simulink model "Controller_ETR"  (R2013b)
settings: Solver=ode45  StartTime=0.0  StopTime=10.0  RelTol=1e-3
undefined symbols (not defined in the file or in its folder): K_dot_track, K_dot_wait, K_track, K_wait
libraries: dspvision x1
settings Model: Creator=hkunte  LastModifiedBy=menkh

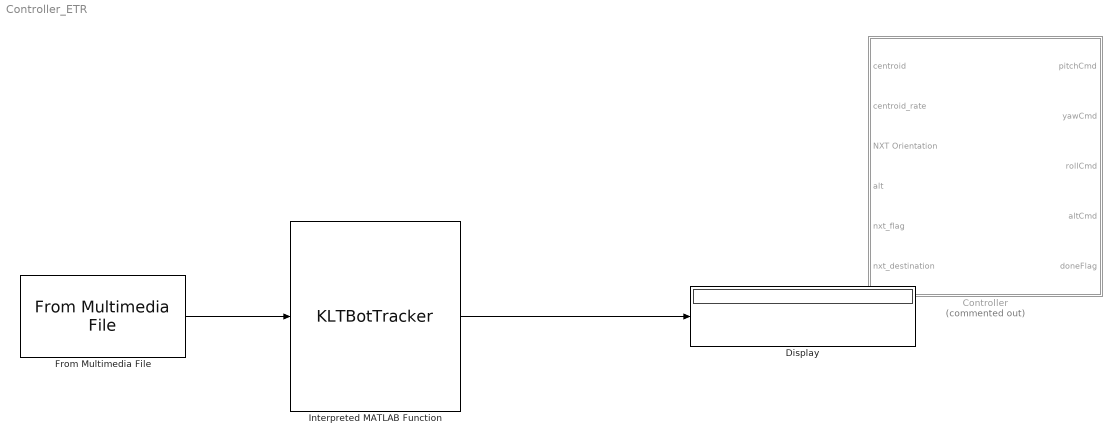
== system Controller_ETR ==
  "Controller " : Subsystem  Commented=on
  Display : Display
  From Multimedia File : dspvision/From Multimedia File  inputFilename=natickTrial7.mp4  loop=on  numPlays=inf  outputStreams=Video only  videoDataType=double  audioDataType=int16  inheritSampleTime=on  userDefinedSampleTime=1/30  noAudioOutput=off  isIntensityVideo=off  fourcc=Intensity  colorVideoFormat=Separate color signals  outputEOF=off  dataOrg=Column-major  audioFrameSize=1024  computeAudioFrameSize=off  outSamplingMode=Sample based
  Interpreted MATLAB Function : MATLABFcn  MATLABFcn=KLTBotTracker  OutputDimensions=[1 2]  Output1D=off
  wires:
  Interpreted MATLAB Function/1 -> Display/1
  From Multimedia File/1 -> Interpreted MATLAB Function/1

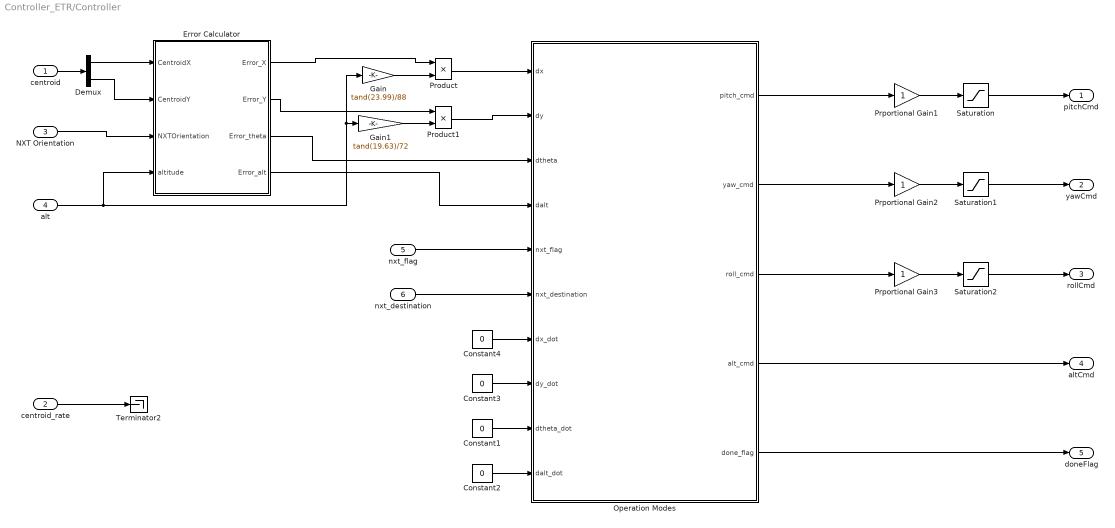
== system Controller_ETR/Controller  ==
  centroid : Inport
  "centroid_rate " : Inport  Port=2  PortDimensions=2
  NXT Orientation : Inport  Port=3
  alt : Inport  Port=4
  nxt_flag : Inport  Port=5  OutDataTypeStr=boolean
  nxt_destination : Inport  Port=6  OutDataTypeStr=boolean
  Constant{1..4} (4 alike) : Constant  Value=0
  Demux : Demux  Outputs=2
  Error Calculator : Subsystem
  Gain : Gain  Gain=tand(23.99)/88
  Gain1 : Gain  Gain=tand(19.63)/72
  Operation Modes : Stateflow chart  TreatAsAtomicUnit=on
  Product : Product
  Product1 : Product
  Prportional Gain1 : Gain
  Prportional Gain2 : Gain
  Prportional Gain3 : Gain
  Saturation : Saturate  UpperLimit=1  LowerLimit=-1
  Saturation1 : Saturate  UpperLimit=1  LowerLimit=-1
  Saturation2 : Saturate  UpperLimit=1  LowerLimit=-1
  Terminator2 : Terminator
  pitchCmd : Outport
  yawCmd : Outport  Port=2
  rollCmd : Outport  Port=3
  altCmd : Outport  Port=4
  doneFlag : Outport  Port=5
  wires:
  Constant2/1 -> Operation Modes/10(dalt_dot)
  Demux/2 -> Error Calculator/2(CentroidY)
  Demux/1 -> Error Calculator/1(CentroidX)
  centroid/1 -> Demux/1
  Saturation1/1 -> yawCmd/1
  Prportional Gain3/1 -> Saturation2/1
  Operation Modes/1(pitch_cmd) -> Prportional Gain1/1
  Saturation2/1 -> rollCmd/1
  Prportional Gain2/1 -> Saturation1/1
  Prportional Gain1/1 -> Saturation/1
  Operation Modes/3(roll_cmd) -> Prportional Gain3/1
  Saturation/1 -> pitchCmd/1
  Operation Modes/2(yaw_cmd) -> Prportional Gain2/1
  Constant3/1 -> Operation Modes/8(dy_dot)
  Constant1/1 -> Operation Modes/9(dtheta_dot)
  Error Calculator/3(Error_theta) -> Operation Modes/3(dtheta)
  Constant4/1 -> Operation Modes/7(dx_dot)
  Product1/1 -> Operation Modes/2(dy)
  Error Calculator/2(Error_Y) -> Product1/1
  Error Calculator/1(Error_X) -> Product/1
  Product/1 -> Operation Modes/1(dx)
  NXT Orientation/1 -> Error Calculator/3(NXTOrientation)
  alt/1 -> Error Calculator/4(altitude), Gain/1, Gain1/1
  Gain/1 -> Product/2
  Gain1/1 -> Product1/2
  nxt_flag/1 -> Operation Modes/5(nxt_flag)
  "centroid_rate "/1 -> Terminator2/1
  nxt_destination/1 -> Operation Modes/6(nxt_destination)
  Operation Modes/5(done_flag) -> doneFlag/1
  Operation Modes/4(alt_cmd) -> altCmd/1
  Error Calculator/4(Error_alt) -> Operation Modes/4(dalt)

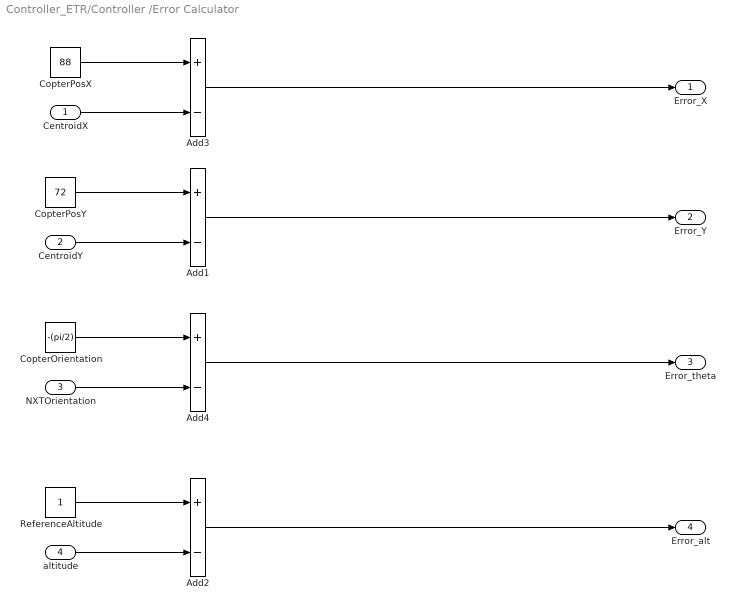
== system Controller_ETR/Controller /Error Calculator ==
  CentroidX : Inport
  CentroidY : Inport  Port=2
  NXTOrientation : Inport  Port=3
  altitude : Inport  Port=4
  Add{1..4} (4 alike) : Sum  Inputs=+-
  CopterOrientation : Constant  Value=-(pi/2)
  CopterPosX : Constant  Value=88
  CopterPosY : Constant  Value=72
  ReferenceAltitude : Constant
  Error_X : Outport
  Error_Y : Outport  Port=2
  Error_theta : Outport  Port=3
  Error_alt : Outport  Port=4
  wires:
  CopterPosY/1 -> Add1/1
  CentroidY/1 -> Add1/2
  CopterPosX/1 -> Add3/1
  CentroidX/1 -> Add3/2
  Add3/1 -> Error_X/1
  Add1/1 -> Error_Y/1
  NXTOrientation/1 -> Add4/2
  CopterOrientation/1 -> Add4/1
  Add4/1 -> Error_theta/1
  ReferenceAltitude/1 -> Add2/1
  altitude/1 -> Add2/2
  Add2/1 -> Error_alt/1

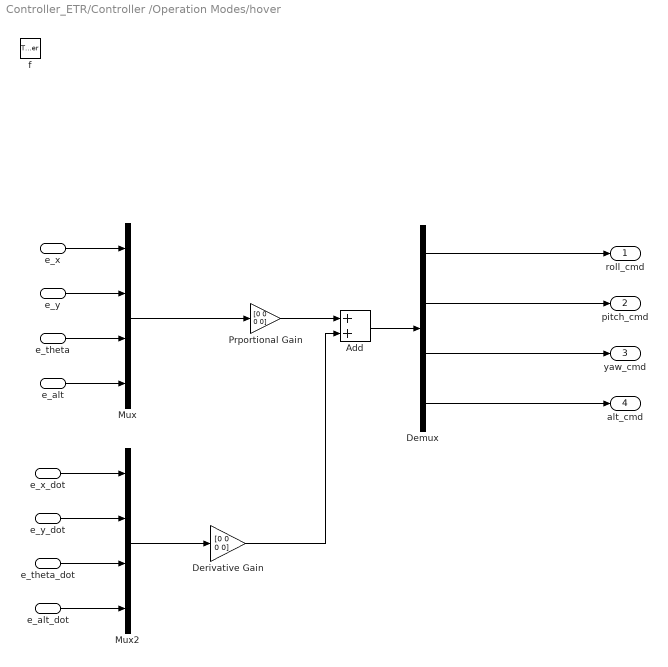
== system Controller_ETR/Controller /Operation Modes/hover ==
  e_x : Inport
  e_y : Inport  Port=2
  e_theta : Inport  Port=3
  e_x_dot : Inport  Port=4
  e_y_dot : Inport  Port=5
  e_theta_dot : Inport  Port=6
  e_alt : Inport  Port=7
  e_alt_dot : Inport  Port=8
  f : TriggerPort  TriggerType=function-call
      settings: CopyFcn=Stateflow.SLINSF.SimulinkMan.removeBlockPreDeleteFcn  PreDeleteFcn=Stateflow.SLINSF.SimulinkMan.unsafePredeleteFcn
  Add : Sum
  Demux : Demux
  Derivative Gain : Gain  Gain=[0 0 0 0]
  Mux : Mux
  Mux2 : Mux
  Prportional Gain : Gain  Gain=[0 0 0 0]
  roll_cmd : Outport
  pitch_cmd : Outport  Port=2
  yaw_cmd : Outport  Port=3
  alt_cmd : Outport  Port=4
  wires:
  Mux/1 -> Prportional Gain/1
  e_x/1 -> Mux/1
  e_y/1 -> Mux/2
  e_theta/1 -> Mux/3
  Prportional Gain/1 -> Add/1
  Derivative Gain/1 -> Add/2
  Add/1 -> Demux/1
  Demux/3 -> yaw_cmd/1
  Demux/1 -> roll_cmd/1
  Demux/2 -> pitch_cmd/1
  Mux2/1 -> Derivative Gain/1
  e_x_dot/1 -> Mux2/1
  e_y_dot/1 -> Mux2/2
  e_theta_dot/1 -> Mux2/3
  e_alt/1 -> Mux/4
  e_alt_dot/1 -> Mux2/4
  Demux/4 -> alt_cmd/1

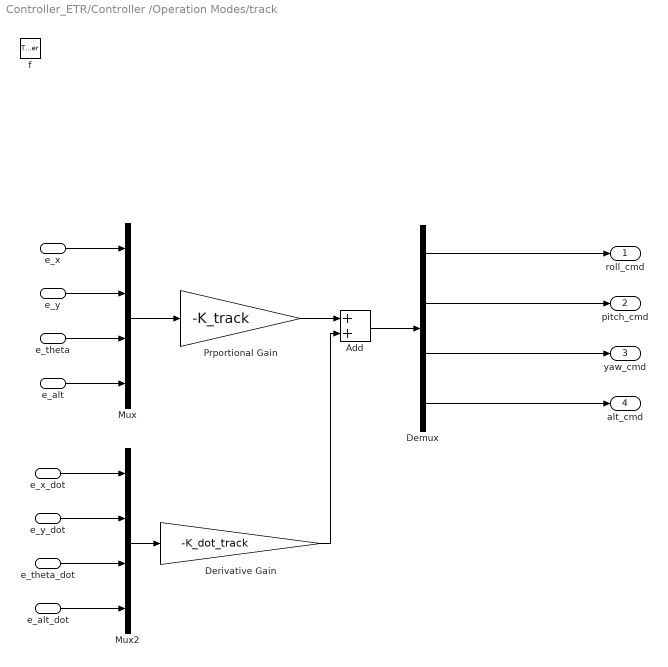
== system Controller_ETR/Controller /Operation Modes/track ==
  e_x : Inport
  e_y : Inport  Port=2
  e_theta : Inport  Port=3
  e_x_dot : Inport  Port=4
  e_y_dot : Inport  Port=5
  e_theta_dot : Inport  Port=6
  e_alt : Inport  Port=7
  e_alt_dot : Inport  Port=8
  f : TriggerPort  TriggerType=function-call
      settings: CopyFcn=Stateflow.SLINSF.SimulinkMan.removeBlockPreDeleteFcn  PreDeleteFcn=Stateflow.SLINSF.SimulinkMan.unsafePredeleteFcn
  Add : Sum
  Demux : Demux
  Derivative Gain : Gain  Gain=-K_dot_track
  Mux : Mux
  Mux2 : Mux
  Prportional Gain : Gain  Gain=-K_track
  roll_cmd : Outport
  pitch_cmd : Outport  Port=2
  yaw_cmd : Outport  Port=3
  alt_cmd : Outport  Port=4
  wires:
  Mux/1 -> Prportional Gain/1
  e_x/1 -> Mux/1
  e_y/1 -> Mux/2
  e_theta/1 -> Mux/3
  Prportional Gain/1 -> Add/1
  Derivative Gain/1 -> Add/2
  Add/1 -> Demux/1
  Demux/3 -> yaw_cmd/1
  Demux/1 -> roll_cmd/1
  Demux/2 -> pitch_cmd/1
  Mux2/1 -> Derivative Gain/1
  e_x_dot/1 -> Mux2/1
  e_y_dot/1 -> Mux2/2
  e_theta_dot/1 -> Mux2/3
  e_alt/1 -> Mux/4
  e_alt_dot/1 -> Mux2/4
  Demux/4 -> alt_cmd/1

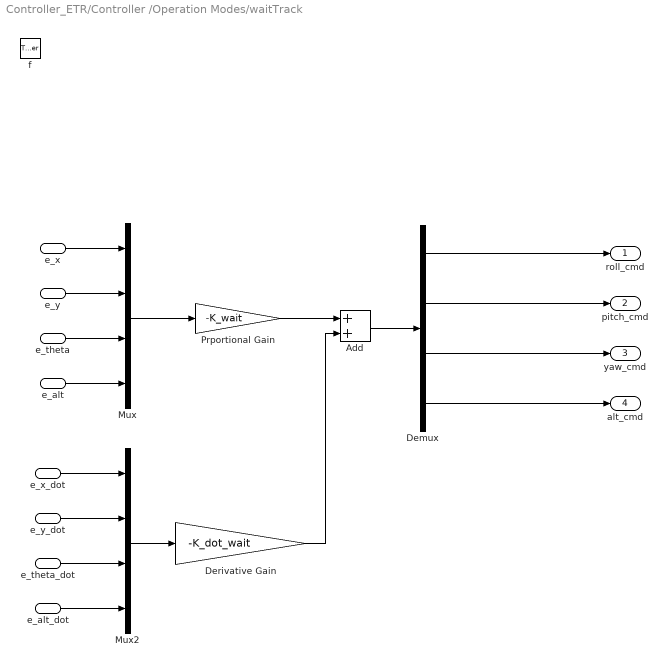
== system Controller_ETR/Controller /Operation Modes/waitTrack ==
  e_x : Inport
  e_y : Inport  Port=2
  e_theta : Inport  Port=3
  e_x_dot : Inport  Port=4
  e_y_dot : Inport  Port=5
  e_theta_dot : Inport  Port=6
  e_alt : Inport  Port=7
  e_alt_dot : Inport  Port=8
  f : TriggerPort  TriggerType=function-call
      settings: CopyFcn=Stateflow.SLINSF.SimulinkMan.removeBlockPreDeleteFcn  PreDeleteFcn=Stateflow.SLINSF.SimulinkMan.unsafePredeleteFcn
  Add : Sum
  Demux : Demux
  Derivative Gain : Gain  Gain=-K_dot_wait
  Mux : Mux
  Mux2 : Mux
  Prportional Gain : Gain  Gain=-K_wait
  roll_cmd : Outport
  pitch_cmd : Outport  Port=2
  yaw_cmd : Outport  Port=3
  alt_cmd : Outport  Port=4
  wires:
  Mux/1 -> Prportional Gain/1
  e_x/1 -> Mux/1
  e_y/1 -> Mux/2
  e_theta/1 -> Mux/3
  Prportional Gain/1 -> Add/1
  Derivative Gain/1 -> Add/2
  Add/1 -> Demux/1
  Demux/3 -> yaw_cmd/1
  Demux/1 -> roll_cmd/1
  Demux/2 -> pitch_cmd/1
  Mux2/1 -> Derivative Gain/1
  e_x_dot/1 -> Mux2/1
  e_y_dot/1 -> Mux2/2
  e_theta_dot/1 -> Mux2/3
  e_alt/1 -> Mux/4
  e_alt_dot/1 -> Mux2/4
  Demux/4 -> alt_cmd/1

== stateflow chart Controller_ETR/Controller /Operation Modes ==
  state InitializeGains
    entry:
    K_wait = [1 1 1 0];
    K_dot_wait = [0 0 0 0];
    K_track = [1 1 1 0];
    K_dot_track = [0 0 0 0];
  state DebugHover
    during:
    [roll_cmd,pitch_cmd,yaw_cmd, alt_cmd] = hover(dx,dy,dtheta,dx_dot,dy_dot,dtheta_dot,dalt,dalt_dot)
  state [roll_cmd,pitch_cmd,yaw_cmd,alt_cmd] = hover(e_x,e_y,e_theta,e_x_dot,e_y_dot,e_theta_dot,e_alt,e_alt_dot) [function]
  state WaitForNXT
    during:
    [roll_cmd,pitch_cmd,yaw_cmd, alt_cmd] = waitTrack(dx,dy,dtheta,dx_dot,dy_dot,dtheta_dot,dalt,dalt_dot)
  state [roll_cmd,pitch_cmd,yaw_cmd,alt_cmd] = waitTrack(e_x,e_y,e_theta,e_x_dot,e_y_dot,e_theta_dot,e_alt,e_alt_dot) [function]
  state NormalTracking
    during:
    [roll_cmd,pitch_cmd,yaw_cmd, alt_cmd] = track(dx,dy,dtheta,dx_dot,dy_dot,dtheta_dot,dalt,dalt_dot)
  state [roll_cmd,pitch_cmd,yaw_cmd,alt_cmd] = track(e_x,e_y,e_theta,e_x_dot,e_y_dot,e_theta_dot,e_alt,e_alt_dot) [function]
  state EndHover
    during:
    done_flag =1
  state FailureHover
    during:
    [roll_cmd,pitch_cmd,yaw_cmd, alt_cmd] = hover(dx,dy,dtheta,dx_dot,dy_dot,dtheta_dot,dalt,dalt_dot)
  (default) -> InitializeGains
  InitializeGains -> DebugHover
  DebugHover -> WaitForNXT : after(30,sec)
  WaitForNXT -> NormalTracking : [nxt_flag ==1]
  NormalTracking -> EndHover [order 2] : [nxt_destination ==1]
  NormalTracking -> FailureHover [order 1] : [nxt_flag ==0]
  FailureHover -> NormalTracking : [nxt_flag==1]
  data: e_x function_input; e_y function_input; e_theta function_input; roll_cmd function_output; pitch_cmd function_output; yaw_cmd function_output; e_x_dot function_input; e_y_dot function_input; e_theta_dot function_input; e_alt function_input; e_alt_dot function_input; alt_cmd function_output; e_x function_input; e_y function_input; e_theta function_input; roll_cmd function_output; pitch_cmd function_output; yaw_cmd function_output; e_x_dot function_input; e_y_dot function_input; e_theta_dot function_input; e_alt function_input; e_alt_dot function_input; alt_cmd function_output; e_x function_input; e_y function_input; e_theta function_input; roll_cmd function_output; pitch_cmd function_output; yaw_cmd function_output; e_x_dot function_input; e_y_dot function_input; e_theta_dot function_input; e_alt function_input; e_alt_dot function_input; alt_cmd function_output; dx input; dy input; dtheta input; pitch_cmd output double; yaw_cmd output double; roll_cmd output double; alt_cmd output double; dalt input; done_flag output boolean; nxt_flag input boolean; nxt_destination input boolean; dx_dot input double; dy_dot input double; dtheta_dot input double; dalt_dot input double; K_wait local double; K_dot_wait local double; K_track local double; K_dot_track local double
